simulink model "pendulo_pv_sem_filtro"  (R2020b)
settings: Solver=FixedStepAuto  StartTime=0.0  StopTime=10  FixedStep=1e-3  RelTol=1e-3
values from neighbouring files (symbols this model uses):
  controlador = projetarControlador(requisitos, planta)    [executarTudo.m]    (also in runAll.m; simular.m)
  planta = obterPlanta()    [codetest.m]    (also in executarTudo.m; nextState.m; runAll.m; simular.m)
  thetar = 0    [executarTudo.m]    (also in runAll.m)
undefined symbols (not defined in the file or in its folder): varCom, varMed
settings Model: Creator=davi  LastModifiedBy=alexandremaranhao

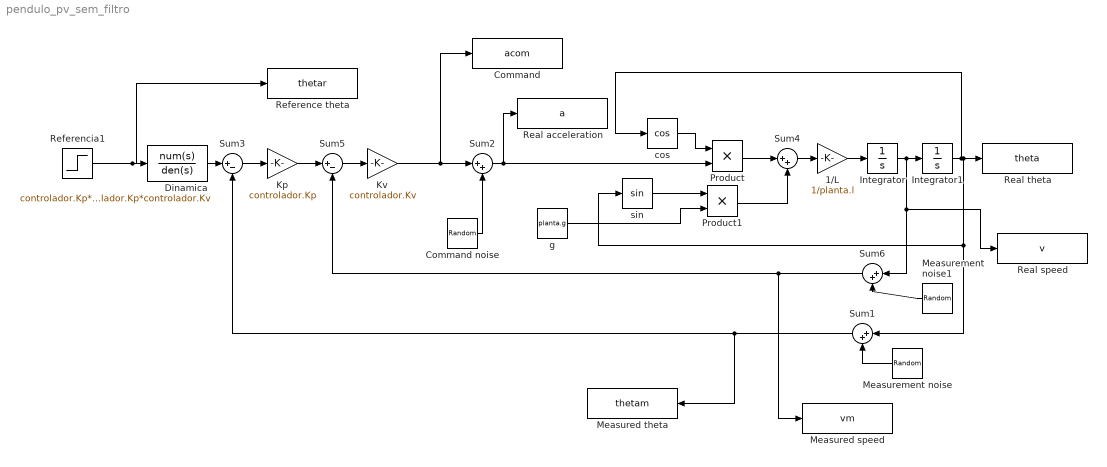
== system pendulo_pv_sem_filtro ==
  1/L : Gain  Gain=1/planta.l
  Command : ToWorkspace  VariableName=acom  SaveFormat=Structure With Time  SampleTime=-1
  Command noise : RandomNumber  Variance=varCom  SampleTime=1e-2
  Dinamica : TransferFcn  Numerator=controlador.Kp*controlador.Kv-planta.g  Denominator=controlador.Kp*controlador.Kv
  Integrator : Integrator
  Integrator1 : Integrator
  Kp : Gain  Gain=controlador.Kp
  Kv : Gain  Gain=controlador.Kv
  Measured speed : ToWorkspace  VariableName=vm  SaveFormat=Structure With Time  SampleTime=-1
  Measured theta : ToWorkspace  VariableName=thetam  SaveFormat=Structure With Time  SampleTime=-1
  Measurement noise : RandomNumber  Variance=varMed  SampleTime=1e-2
  Measurement noise1 : RandomNumber  Variance=varMed  SampleTime=1e-2
  Product : Product
  Product1 : Product
  Real acceleration : ToWorkspace  VariableName=a  SaveFormat=Structure With Time  SampleTime=-1
  Real speed : ToWorkspace  VariableName=v  SaveFormat=Structure With Time  SampleTime=-1
  Real theta : ToWorkspace  VariableName=theta  SaveFormat=Structure With Time  SampleTime=-1
  Reference theta : ToWorkspace  VariableName=thetar  SaveFormat=Structure With Time  SampleTime=-1
  Referencia1 : Step  Time=0  After=thetar  SampleTime=0
  Sum{1..2,4,6} (4 alike) : Sum  Inputs=|++
  Sum3 : Sum  Inputs=|+-
  Sum5 : Sum  Inputs=|+-
  cos : Trigonometry  Operator=cos
  g : Constant  Value=planta.g
  sin : Trigonometry
  wires:
  Product/1 -> Sum4/1
  Measurement noise/1 -> Sum1/2
  Sum2/1 -> Product/2, Real acceleration/1
  Command noise/1 -> Sum2/2
  Referencia1/1 -> Reference theta/1, Dinamica/1
  cos/1 -> Product/1
  sin/1 -> Product1/1
  g/1 -> Product1/2
  Product1/1 -> Sum4/2
  Sum4/1 -> 1/L/1
  1/L/1 -> Integrator/1
  Integrator/1 -> Sum6/1, Real speed/1, Integrator1/1
  Integrator1/1 -> sin/1, Sum1/1, Real theta/1, cos/1
  Sum3/1 -> Kp/1
  Sum6/1 -> Sum5/2, Measured speed/1
  Sum1/1 -> Sum3/2, Measured theta/1
  Kv/1 -> Command/1, Sum2/1
  Kp/1 -> Sum5/1
  Sum5/1 -> Kv/1
  Measurement noise1/1 -> Sum6/2
  Dinamica/1 -> Sum3/1
